simulink library "heat_exchanger_storage"  (R2018b)
settings: Solver=ode45  StartTime=0.0  StopTime=10.0  RelTol=1e-3  EnableMultiTasking=on
libraries: carnot x4
settings Model: Creator=lena.frank  LastModifiedBy=drhf
settings DataIOCC: LimitDataPoints=on  SaveFormat=Array  SignalLoggingSaveFormat=ModelDataLogs
settings OptimizationCC: ExpressionDepthLimit=2147483647  LifeSpan=inf
settings DebuggingCC: UnderspecifiedInitializationDetection=Classic  MergeDetectMultiDrivingBlocksExec=none  SolverPrmCheckMsg=warning  FcnCallInpInsideContextMsg=warning  StateNameClashWarn=warning  SFUnexpectedBacktrackingDiag=warning  SFNoUnconditionalDefaultTransitionDiag=warning  SFExecutionAtInitializationDiag=none
settings HardwareCC: ProdBitPerPointer=32  ProdBitPerSizeT=32  ProdBitPerPtrDiffT=32  ProdLargestAtomicFloat=None  ProdIntDivRoundTo=Undefined  ProdEndianess=Unspecified  ProdWordSize=32  ProdHWDeviceType=32-bit Generic
settings ModelReferenceCC: PropagateSignalLabelsOutOfModel=off
settings SFSimCC: SimUseLocalCustomCode=off
settings RTWCC: RTWUseLocalCustomCode=off
settings CodeAppCC: StateflowObjectComments=on
settings GRTTargetCC: TargetLangStandard=C89/C90 (ANSI)  GeneratePreprocessorConditionals=Disable all  CombineOutputUpdateFcns=off  GRTInterface=on
settings ConfigComp: CovMetricSettings=dw  CovHtmlReporting=on  CovSaveCumulativeToWorkspaceVar=on  CovSaveSingleToWorkspaceVar=on  CovExternalEMLEnable=off

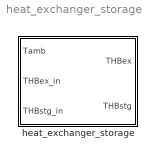
== system heat_exchanger_storage ==
  heat_exchanger_storage : Subsystem  mask(storage with heat exchanger){v=[0.002 0.0005], loss=0.1, uh=[500 1], uc=[500 1], uw=[300 1], mat=aluminium, m=[3 0.1], t0=20, dph=[200 100 1], dpc=[20 10 0.5], n=1}
      mask prompts: v "volume [exchanger storage] [m³]"; loss "ua losses [W/K]"; uh "heat transfer in exchanger [constant linear_in_massflow] [W/K]"; uc "heat transfer to storage [constant linear_massflow] [W/K]"; uw "heat transfer to wall [constant linear_in_massflow] [W/K]"; mat "material"; m "[mass_in_kg fraction_exchanger]"; t0 "initial temperature [degree centigrade]"; dph "pressure drop exchanger [linear quadratic lin_T] [Pa]"; dpc "pressure drop storage [linear quadratic lin_T] [Pa]"; n "number of nodes"
      mask help: This block is a heat exchanger, taking the fluid volume of the cold and hot side and the thermal capacity of the walls into account.
      mask init:
      | v = max(0.00001, v);
      | n = max(n,1);
      mask Help: web(fullfile(path_carnot('help'),'heat_exchanger_storage.html'),'-helpbrowser')
      mask TypeOptions mat: aluminium | bronze | cast iron | steel | stainless steel | copper | brass | gravel | granite | glass | PU-foam | glass wool
      mask Display: plot(0,-10,110,95,[30,30,35,65,70,70,65,35,30],[90,60,54,54,60,90,95,95,90],[30,66,34,66,34,66,30],[63,63,68,73,76,81,81])

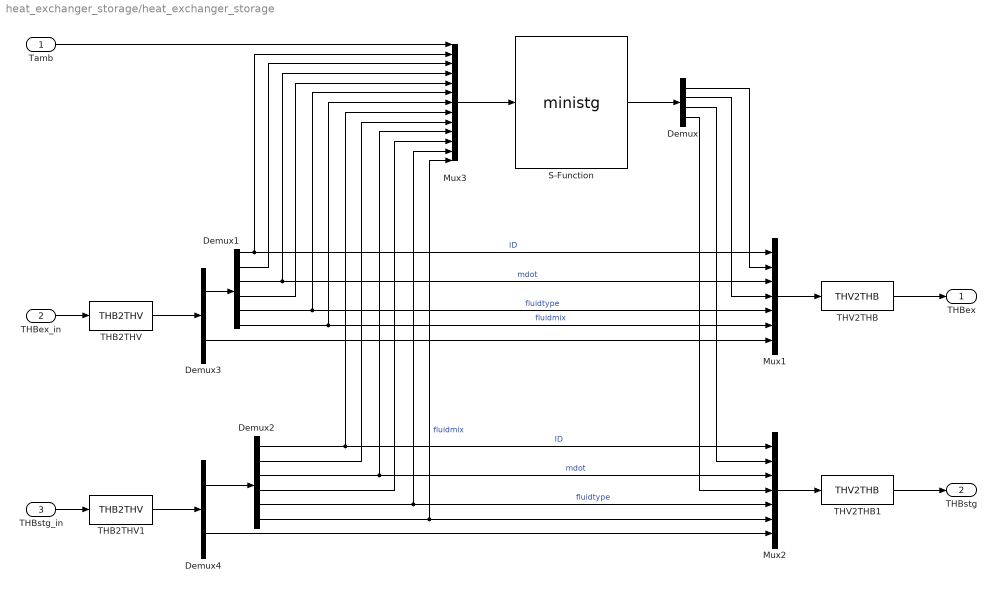
== system heat_exchanger_storage/heat_exchanger_storage ==
  Tamb : Inport
  THBex_in : Inport  Port=2
  THBstg_in : Inport  Port=3
  Demux : Demux
  Demux1 : Demux  Outputs=[1 1 1 1 1 1]
  Demux2 : Demux  Outputs=[1 1 1 1 1 1]
  Demux3 : Demux  Outputs=[6 14]
  Demux4 : Demux  Outputs=[6 14]
  Mux1 : Mux  Inputs=7
  Mux2 : Mux  Inputs=7
  Mux3 : Mux  Inputs=13
  S-Function : S-Function  FunctionName=ministg  Parameters=v(1), v(2), loss, uh(1), uh(2), uc(1), uc(2), uw(1), uw(2), mat, m(1), m(2), t0, dph(1), dph(2), dph(3), dpc(1), dpc(2), dpc(3), n  SFunctionDeploymentMode=off  EnableBusSupport=off
  THB2THV : carnot/Toolbox/THB2THV
      settings: SourceProductName=Carnot
  THB2THV1 : carnot/Toolbox/THB2THV
      settings: SourceProductName=Carnot
  THV2THB : carnot/Toolbox/THV2THB
      settings: SourceProductName=Carnot
  THV2THB1 : carnot/Toolbox/THV2THB
      settings: SourceProductName=Carnot
  THBex : Outport
  THBstg : Outport  Port=2
  wires:
  Demux4/2 -> Mux2/7
  Demux3/2 -> Mux1/7
  Demux/1 -> Mux1/2
  Demux/2 -> Mux1/4
  Mux1/1 -> THV2THB/1
  Mux2/1 -> THV2THB1/1
  Demux/3 -> Mux2/2
  Demux/4 -> Mux2/4
  Demux4/1 -> Demux2/1
  THBstg_in/1 -> THB2THV1/1
  THBex_in/1 -> THB2THV/1
  Demux3/1 -> Demux1/1
  S-Function/1 -> Demux/1
  Demux2/1 -> Mux3/8, Mux2/1  "ID"
  Demux2/2 -> Mux3/9
  Demux2/4 -> Mux3/11
  Demux1/1 -> Mux3/2, Mux1/1  "ID"
  Tamb/1 -> Mux3/1
  Demux1/2 -> Mux3/3
  Demux1/4 -> Mux3/5
  Demux1/3 -> Mux3/4, Mux1/3  "mdot"
  Demux1/5 -> Mux3/6, Mux1/5  "fluidtype"
  Demux2/3 -> Mux3/10, Mux2/3  "mdot"
  Demux2/5 -> Mux3/12, Mux2/5  "fluidtype"
  THB2THV/1 -> Demux3/1
  THB2THV1/1 -> Demux4/1
  THV2THB/1 -> THBex/1
  THV2THB1/1 -> THBstg/1
  Demux1/6 -> Mux3/7, Mux1/6  "fluidmix"
  Demux2/6 -> Mux3/13, Mux2/6  "fluidmix"
  Mux3/1 -> S-Function/1
